simulink model "control_adaptativo"  (R2020b)
settings: Solver=ode45  StartTime=0.0  StopTime=50  FixedStep=0.02  RelTol=1e-3
settings Model: Creator=Dhilan  LastModifiedBy=Marco

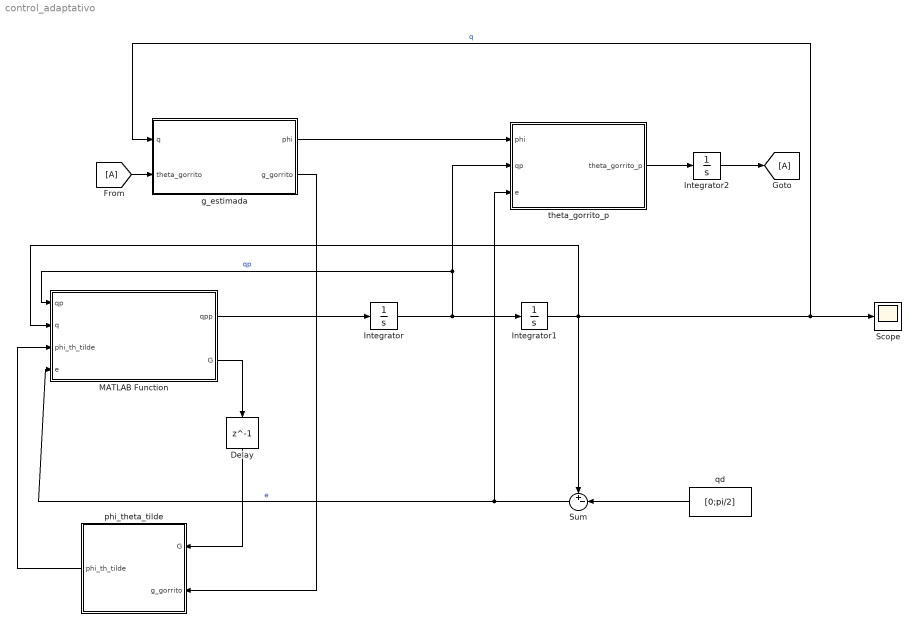
== system control_adaptativo ==
  Delay : Delay  DelayLength=1
  Integrator : Integrator  InitialCondition=[0;0]
  Integrator1 : Integrator  InitialCondition=[0;0]
  Integrator2 : Integrator  InitialCondition=[0.1;0.1;0.1]
  MATLAB Function : MATLAB Function  TreatAsAtomicUnit=on
  Scope : Scope
  Sum : Sum  Inputs=+-|
  g_estimada : MATLAB Function  TreatAsAtomicUnit=on
  phi_theta_tilde : MATLAB Function  TreatAsAtomicUnit=on
  qd : Constant  Value=[0;pi/2]  VectorParams1D=off
  theta_gorrito_p : MATLAB Function  TreatAsAtomicUnit=on
  wires:
  g_estimada/2(g_gorrito) -> phi_theta_tilde/2(g_gorrito)
  MATLAB Function/1(qpp) -> Integrator/1
  Integrator/1 -> MATLAB Function/1(qp), theta_gorrito_p/2(qp), Integrator1/1  "qp"
  Integrator1/1 -> MATLAB Function/2(q), Sum/1, g_estimada/1(q), Scope/1  "q"
  Sum/1 -> theta_gorrito_p/3(e), MATLAB Function/4(e)  "e"
  g_estimada/1(phi) -> theta_gorrito_p/1(phi)
  MATLAB Function/2(G) -> Delay/1
  theta_gorrito_p/1(theta_gorrito_p) -> Integrator2/1
  [A] -> g_estimada/2(theta_gorrito)
  phi_theta_tilde/1(phi_th_tilde) -> MATLAB Function/3(phi_th_tilde)
  Integrator2/1 -> [A]
  Delay/1 -> phi_theta_tilde/1(G)
  qd/1 -> Sum/2

== matlab function control_adaptativo/g_estimada ==
  data: phi output; q input; g_gorrito output; theta_gorrito input
function [phi,g_gorrito]  = fcn(q,theta_gorrito)

g = 9.8; %m/s2

phi = [g*cos(q(1)) g*cos(q(1)+q(2))  g*cos(q(1));
             0 g*cos(q(1)+q(2)) 0];
% theta_gorrito = [m1*lc1; m2*lc2; m2*lc2]; 

g_gorrito = phi*theta_gorrito;

== matlab function control_adaptativo/MATLAB Function ==
  data: qp input; q input; phi_th_tilde input; qpp output; G output; e input
function [qpp,G] = fcn(qp,q,phi_th_tilde,e)
%ganacias de control
% kd = [0.55 0;0 0.9];
% kp = [0.1 0;0 0.1];
kd = [2.4 0;0 3.3];
kp = [1 0;0 1];
%Parametros reales del robot b1
% I1 = 0.5; %kgm2
% m1 = 0.5; %kg
% l1 = 0.5; %m
% lc1 = l1/2; %m
% I2 = 0.3; %kmg2
% m2 = 0.3; %kg
% l2 = 0.3; %m
% lc2 = l2/2; %m
% g = 9.8; %m/s2

%Parametros reales del robot b2
I1 = 0.5; %kgm2
m1 = 0.5; %kg
l1 = 0.5; %m
lc1 = l1/2; %m
I2 = 0.3; %kmg2
m2 = 0.3; %kg
l2 = 0.3; %m
lc2 = l2/2; %m
g = 9.8; %m/s2

% Matriz de inercia
M11 = m1*lc1^2 + I1 + m2*(l1^2 + lc2^2 + 2*l1*lc2*cos(q(2))) + I2;
M22 = m2*lc2^2 + I2;
M12 = m2*l1*lc2*cos(q(2)) + m2*lc2^2 + I2;
M = [M11 M12; M12 M22];

% Matriz de coriolis
C11 = -(m2*l1*lc2*sin(q(2)))*qp(2);
C12 = -(m2*l1*lc2*sin(q(2)))*qp(1) + C11;
C21 = (m2*l1*lc2*sin(q(2)))*qp(1);
C = [C11 C12;C21 0];

% Vector de gravedad
g1 = m1*lc1*g*cos(q(1)) + m2*g*(lc2*cos(q(1) + q(2)) + l1*cos(q(1)));
g2 = m2*g*lc2*cos(q(1)+q(2));
G = [g1;g2];

%-phi_th_tilde para que se vuelva positiva
qpp = M\(-C*qp+phi_th_tilde-kp*e-kd*qp);

== matlab function control_adaptativo/phi_theta_tilde ==
  data: G input; g_gorrito input; phi_th_tilde output
function phi_th_tilde = fcn(G,g_gorrito)

phi_th_tilde = -(G-g_gorrito);

== matlab function control_adaptativo/theta_gorrito_p ==
  data: phi input; theta_gorrito_p output; qp input; e input
function theta_gorrito_p = fcn(phi,qp,e)
T = [5 0 0;0 5 0; 0 0 5];
gamma = 0.3;
theta_gorrito_p = -T*(phi')*(qp(:)+ (gamma.*[tanh(e(1));tanh(e(2))]));
